simulink model "BD_PAR_SA"  (Simulink 4.1.1)
settings: Solver=ode1  SolverMode=SingleTasking  StartTime=0.0  StopTime=max(cyc_mph(:,1))  FixedStep=1  MaxStep=1  RelTol=1e-3  AbsTol=1e-3
undefined symbols (not defined in the file): ess_on, ex_calc, fc_emis, fc_max_trq, fc_trq_scale, mc_max_trq, mc_overtrq_factor, mc_trq_scale, vc_idle_spd
libraries: lib_transmission x4, lib_wheel x2, lib_controls x2, lib_help x2, lib_accessory x2, lib_outputs x1, lib_interactive x1, lib_drive_cycle x1, lib_energy_storage x1, lib_exhaust x1, lib_fuel_converter x1, lib_electric_machine x1
settings Model: LastModifiedBy=ssprik  ModifiedComment=ssprik -- Wed Sep 24 15:09:53 2003 -- Version 1.36  SaveTime=off  SaveOutput=off  LimitDataPoints=off  UnconnectedLineMsg=none  RTWTemplateMakefile=grt_vc.tmf  ExtModeTrigMode=oneshot  ExtModeArmWhenConnect=off
settings Model: ModifiedHistory=|
  | ssprik -- Wed Sep 24 15:09:53 2003 -- Version 1.36
  | 
  | 
  | abrooker -- Mon Feb 10 13:03:17 2003 -- Version 1.35
  | added altia block for dynamic graphics
  | 
  | mokeefe -- Fri Aug 30 07:47:36 2002 -- Version 1.34
  | Changed the input to "mechanical accessory loads <acc>/Mechanical Accessory Loads V2 <acc>" masked parameter input blocks. In R13, the function "not" no longer returns double 1 or double 0 for true and false but instead returns type logical (boolean). Thus, I am now multiplying by double 1 which causes a type conversion to double yielding the desired effect.
  | 
  | 
  | abrooker -- Tue May 14 11:46:29 2002 -- Version 1.33
  | 
  | 
  | mokeefe -- Thu Apr 18 08:03:37 2002 -- Version 1.32
  | saving the model:
  | o "without the model browser open"
  | o with only top-level screen visible
  | o and with "fit to view" enabled

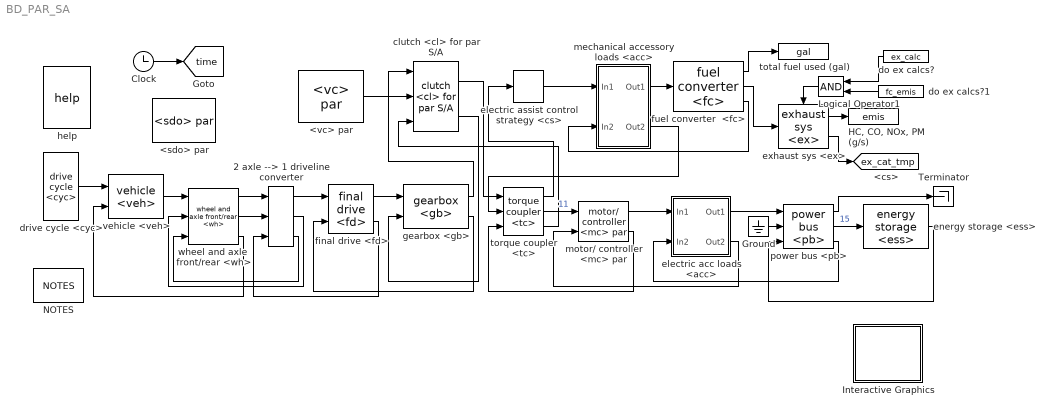
== system BD_PAR_SA ==
  2 axle --> 1 driveline converter : lib_wheel/2 axle --> 1 driveline converter
      settings: RTWFcnNameOpts=Auto  RTWFileNameOpts=Auto
  <sdo> par : lib_outputs/<sdo> par
  <vc> par : lib_controls/<vc> par
      link override config traction control: BlockChoice=traction control
  Clock : Clock
      settings: DisplayTime=off  Decimation=10
  Ground : Ground
  "HC, CO, NOx, PM (g/s)" : ToWorkspace  VariableName=emis  SampleTime=0  SaveFormat=Array
  Interactive Graphics : Subsystem  BlockChoice=off
      settings: AttributesFormatString=%<BlockChoice>  TemplateBlock=lib_interactive/Interactive Graphics  MemberBlocks=off,on  RTWFcnNameOpts=Auto  RTWFileNameOpts=Auto
  Logical Operator1 : Logic  Orientation=left  Operator=AND  Inputs=2
  NOTES : lib_help/NOTES
  Terminator : Terminator
  clutch <cl> for par S/A : lib_transmission/clutch <cl> for par S//A  slip_spd=vc_launch_spd  maxtrq=max(fc_max_trq)*fc_trq_scale+max(mc_max_trq)*mc_overtrq_factor*mc_trq_scale
  do ex calcs? : Constant  Orientation=left  Value=ex_calc
  do ex calcs?1 : Constant  Orientation=left  Value=fc_emis
  drive cycle <cyc> : lib_drive_cycle/drive cycle <cyc>
  electric acc loads <acc> : Subsystem
      settings: RTWFcnNameOpts=Auto  RTWFileNameOpts=Auto
      mask Display: image(imread('bdi_acc_elec.bmp'))
  electric assist control strategy <cs> : lib_controls/electric assist control strategy <cs>
  energy storage <ess> : lib_energy_storage/energy storage <ess>  AncestorBlock=lib_energy_storage/Subsystem/energy storage <ess>
  exhaust sys <ex> : lib_exhaust/exhaust sys <ex>
  final drive <fd> : lib_transmission/final drive <fd>
  fuel converter  <fc> : lib_fuel_converter/fuel converter  <fc>
  gearbox <gb> : lib_transmission/gearbox <gb>
  help : lib_help/help
  mechanical accessory loads <acc> : Subsystem
      settings: RTWFcnNameOpts=Auto  RTWFileNameOpts=Auto
      mask Display: image(imread('bdi_acc_pic.bmp'))
  motor/ controller <mc> par : lib_electric_machine/motor// controller <mc> par
  power bus <pb> : lib_power_bus/power bus <pb>
  torque coupler <tc> : lib_transmission/torque coupler <tc>
  total fuel used (gal) : ToWorkspace  VariableName=gal  SampleTime=0  SaveFormat=Array
  vehicle <veh> : lib_vehicle/vehicle <veh>
      link override rolling resistance force: BlockChoice=force req'd to overcome rolling resistance (N)
      link override vehicle speed: BlockChoice=vehicle speed (m/s)
  wheel and axle  front/rear <wh> : lib_wheel/wheel and axle  front//rear <wh>
  tag scope: ex_cat_tmp=global, time=global
  wires:
  final drive <fd>/1 -> gearbox <gb>/1
  drive cycle <cyc>/1 -> vehicle <veh>/1
  fuel converter  <fc>/2 -> exhaust sys <ex>/1
  do ex calcs?/1 -> Logical Operator1/1
  fuel converter  <fc>/1 -> total fuel used (gal)/1
  exhaust sys <ex>/1 -> "HC, CO, NOx, PM (g/s)"/1
  Logical Operator1/1 -> exhaust sys <ex>/Enable
  do ex calcs?1/1 -> Logical Operator1/2
  Clock/1 -> [time]
  gearbox <gb>/2 -> final drive <fd>/2
  torque coupler <tc>/2 -> motor/ controller <mc> par/1  "11"
  <vc> par/1 -> clutch <cl> for par S/A/2
  motor/ controller <mc> par/2 -> torque coupler <tc>/3
  Ground/1 -> power bus <pb>/2
  power bus <pb>/2 -> energy storage <ess>/1  "15"
  power bus <pb>/1 -> Terminator/1
  energy storage <ess>/1 -> power bus <pb>/3
  gearbox <gb>/1 -> clutch <cl> for par S/A/1
  clutch <cl> for par S/A/2 -> gearbox <gb>/2
  clutch <cl> for par S/A/1 -> torque coupler <tc>/1
  torque coupler <tc>/1 -> electric assist control strategy <cs>/1
  torque coupler <tc>/3 -> clutch <cl> for par S/A/3
  exhaust sys <ex>/2 -> [ex_cat_tmp]
  motor/ controller <mc> par/1 -> electric acc loads <acc>/1(In1)
  electric acc loads <acc>/1(Out1) -> power bus <pb>/1
  power bus <pb>/3 -> electric acc loads <acc>/2(In2)
  electric acc loads <acc>/2(Out2) -> motor/ controller <mc> par/2
  electric assist control strategy <cs>/1 -> mechanical accessory loads <acc>/1(In1)
  mechanical accessory loads <acc>/1(Out1) -> fuel converter  <fc>/1
  fuel converter  <fc>/3 -> mechanical accessory loads <acc>/2(In2)
  mechanical accessory loads <acc>/2(Out2) -> torque coupler <tc>/2
  vehicle <veh>/1 -> wheel and axle  front/rear <wh>/1
  wheel and axle  front/rear <wh>/1 -> 2 axle --> 1 driveline converter/1
  wheel and axle  front/rear <wh>/2 -> 2 axle --> 1 driveline converter/2
  2 axle --> 1 driveline converter/1 -> final drive <fd>/1
  2 axle --> 1 driveline converter/2 -> wheel and axle  front/rear <wh>/2
  2 axle --> 1 driveline converter/3 -> wheel and axle  front/rear <wh>/3
  wheel and axle  front/rear <wh>/3 -> vehicle <veh>/2
  final drive <fd>/2 -> 2 axle --> 1 driveline converter/3

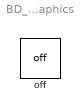
== system BD_PAR_SA/Interactive Graphics ==
  off : lib_interactive/off  Tag=Altia_off  Orientation=up

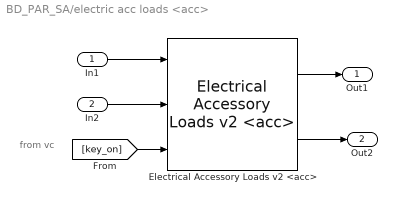
== system BD_PAR_SA/electric acc loads <acc> ==
  note: from vc
  In1 : Inport  Port=1  LatchInput=off
  In2 : Inport  Port=2  LatchInput=off
  Electrical Accessory Loads v2 <acc> : lib_accessory/Electrical Accessory Loads v2 <acc>  load_on=ess_on
      link override backward model/electrical accessories (W): BlockChoice=Electrical Accessories: Time Variable
  Out1 : Outport  Port=1
  Out2 : Outport  Port=2
  wires:
  In1/1 -> Electrical Accessory Loads v2 <acc>/1
  In2/1 -> Electrical Accessory Loads v2 <acc>/2
  Electrical Accessory Loads v2 <acc>/1 -> Out1/1
  Electrical Accessory Loads v2 <acc>/2 -> Out2/1
  [key_on] -> Electrical Accessory Loads v2 <acc>/3

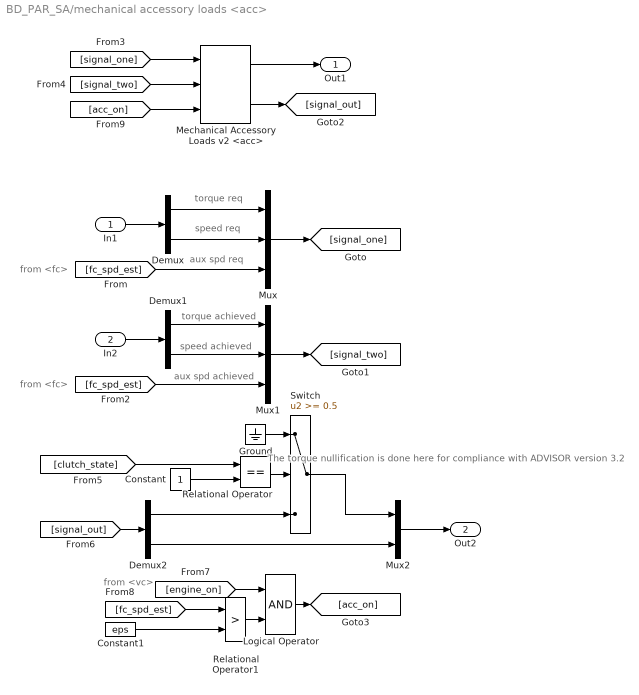
== system BD_PAR_SA/mechanical accessory loads <acc> ==
  note: from <fc>
  note: from <fc>
  note: torque req
  note: speed req
  note: aux spd req
  note: torque achieved
  note: speed achieved
  note: aux spd achieved
  note: The torque nullification is done here for
      | compliance with ADVISOR version 3.2
  note: from <vc>
  In1 : Inport  Port=1  LatchInput=off
  In2 : Inport  Port=2  LatchInput=off
  Constant : Constant  Value=1
  Constant1 : Constant  Value=eps
  Demux : Demux  Outputs=2  BusSelectionMode=off
  Demux1 : Demux  Outputs=2  BusSelectionMode=off
  Demux2 : Demux  Outputs=2  BusSelectionMode=off
  Ground : Ground
  Logical Operator : Logic  Operator=AND  Inputs=2
  Mechanical Accessory Loads v2 <acc> : lib_accessory/Mechanical Accessory Loads v2 <acc>  load_on=not(ess_on)*1  acc_max_spd=inf  acc_min_spd=vc_idle_spd+eps  ic_mech_trq=0  ic_mech_pwr=0
      link override backward model/mechanical accessories (Nm): BlockChoice=Mechanical Accessories: Const Mech Var Elect
      link override estimated mechanical torque/mechanical accessories (Nm): BlockChoice=Mechanical Accessories: Const Mech Var Elect
  Mux : Mux  Inputs=3
  Mux1 : Mux  Inputs=3
  Mux2 : Mux  Inputs=2
  Relational Operator : RelationalOperator  Operator===
  Relational Operator1 : RelationalOperator  Operator=>
  Switch : Switch  Threshold=0.5
  Out1 : Outport  Port=1
  Out2 : Outport  Port=2
  wires:
  [signal_one] -> Mechanical Accessory Loads v2 <acc>/1
  Mechanical Accessory Loads v2 <acc>/1 -> Out1/1
  Mechanical Accessory Loads v2 <acc>/2 -> [signal_out]
  [signal_two] -> Mechanical Accessory Loads v2 <acc>/2
  [acc_on] -> Mechanical Accessory Loads v2 <acc>/3
  Mux/1 -> [signal_one]
  In1/1 -> Demux/1
  Demux/1 -> Mux/1
  Demux/2 -> Mux/2
  [fc_spd_est] -> Mux/3
  Mux1/1 -> [signal_two]
  In2/1 -> Demux1/1
  Demux1/1 -> Mux1/1
  Demux1/2 -> Mux1/2
  [fc_spd_est] -> Mux1/3
  Mux2/1 -> Out2/1
  [clutch_state] -> Relational Operator/1
  Constant/1 -> Relational Operator/2
  Ground/1 -> Switch/1
  Relational Operator/1 -> Switch/2
  [signal_out] -> Demux2/1
  Demux2/2 -> Mux2/2
  Demux2/1 -> Switch/3
  Switch/1 -> Mux2/1
  [fc_spd_est] -> Relational Operator1/1
  Constant1/1 -> Relational Operator1/2
  [engine_on] -> Logical Operator/1
  Relational Operator1/1 -> Logical Operator/2
  Logical Operator/1 -> [acc_on]
